simulink model "eVTOL_System"  (R2024b)
settings: Solver=FixedStepAuto  StartTime=0.0  StopTime=inf  RelTol=1e-3
undefined symbols (not defined in the file): airspeed, Battery, BCE12, BCE_Set_init, BMS_Controller_State, C, Cell10_P, Cell11_P, Cell12_P, Cell13_P, Cell14_P, Cell15_P, Cell16_P, Cell17_P, Cell18_P, Cell19_P, Cell1_N, Cell1_P, Cell20_P, Cell21_P, Cell22_P, Cell23_P, Cell24_P, Cell2_P, Cell3_P, Cell4_P, Cell5_P, Cell6_P, Cell7_P, Cell8_P, Cell9_P, Charging_State, CityMission, control, controlParams, ControlSampleTime, CriticalTiltAngle, currentFactor, CV_Gain, ddx, ddy, ddz, Device_01, Device_02, DiscIntNeverNeededParam, dx, dy, dz, Earth, env, F, F28379D_ADC_MaxCount, F28379D_ADC_Vmax, FixedWingMission, flightState, Foc_Ki_IxTcpu, Foc_Ki_S, Foc_Kp_I, Foc_Kp_S, fractalcoef ... (+68)
libraries: fl_lib x1115, nesl_utility x617, slrealtimeethercatlib x217, simulink x130, canmsglib x101, speedgoatlib_IO611_obsolete x91, slpidlib x49, mcbcontrolslib x44, slrealtimeutilitieslib x35, speedgoatlib_hdlCoder_IO3xx x31, dspstat3 x24, mcbpositiondecoderlib x12
(part 16 of 31)

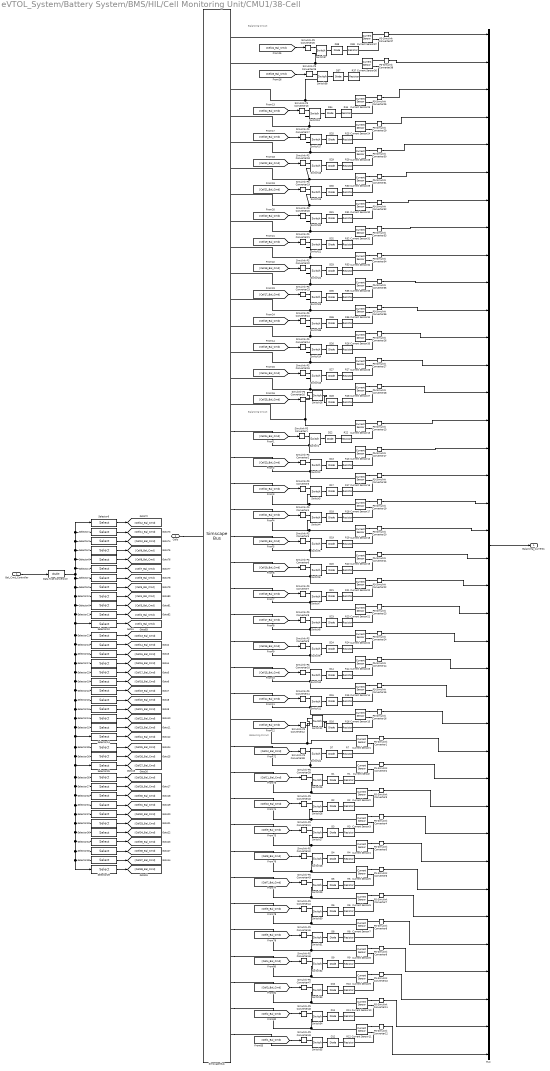
== system eVTOL_System/Battery System/BMS/HIL/Cell Monitoring Unit/CMU1/38-Cell ==
  note: Balancing Circuit
  note: Balancing Circuit
  note: Balancing Circuit
  Bal_Cmd_Controller : Inport
  Current Sensor{,1..37} (38 alike) : fl_lib/Electrical/Electrical Sensors/Current Sensor
  D{1..38} (38 alike) : fl_lib/Electrical/Electrical Elements/Diode  Vf=0.6 V  Ron=0.3 Ohm  Goff=1e-8 1/Ohm  i_specify=off  i_priority=High  i=0 A  i_nominal_specify=off  i_nominal_value=1  i_nominal_unit=A  v_specify=off  v_priority=None  v=0 V  v_nominal_specify=off  v_nominal_value=1  v_nominal_unit=V
      settings: LibrarySourceBlock=BatteryPack_lib/CellMonitoringUnit/D1  LogSimulationData=on
  Data Type Conversion : DataTypeConversion  OutDataTypeStr=double  SaturateOnIntegerOverflow=off  RndMeth=Floor
  Mux : Mux  Inputs=38
  PS-Simulink Converter{1..38} (38 alike) : nesl_utility/PS-Simulink Converter  PhysicalDomain=network_engine_domain  SubClassName=ps_output  LeftPortType=input  RightPortType=output  PseudoPeriodic=off  Frequencies=[]  VectorFormat=inherit  Unit=inherit  AffineConversion=off
  R{1..38} (38 alike) : fl_lib/Electrical/Electrical Elements/Resistor  R=Battery.R_bleed Ohm  i_specify=off  i_priority=None  i=0 A  i_nominal_specify=off  i_nominal_value=1  i_nominal_unit=A  v_specify=off  v_priority=None  v=0 V  v_nominal_specify=off  v_nominal_value=1  v_nominal_unit=V
      settings: LibrarySourceBlock=BatteryPack_lib/CellMonitoringUnit/R1  LogSimulationData=on
  Selector1 : Selector  IndexOptions=Index vector (dialog)  Indices=11  OutputSizes=1
  Selector10 : Selector  IndexOptions=Index vector (dialog)  Indices=1  OutputSizes=1
  Selector11 : Selector  IndexOptions=Index vector (dialog)  Indices=2  OutputSizes=1
  Selector12 : Selector  IndexOptions=Index vector (dialog)  Indices=4  OutputSizes=1
  Selector13 : Selector  IndexOptions=Index vector (dialog)  Indices=14  OutputSizes=1
  Selector14 : Selector  IndexOptions=Index vector (dialog)  Indices=24  OutputSizes=1
  Selector15 : Selector  IndexOptions=Index vector (dialog)  Indices=23  OutputSizes=1
  Selector16 : Selector  IndexOptions=Index vector (dialog)  Indices=21  OutputSizes=1
  Selector17 : Selector  IndexOptions=Index vector (dialog)  Indices=16  OutputSizes=1
  Selector18 : Selector  IndexOptions=Index vector (dialog)  Indices=15  OutputSizes=1
  Selector19 : Selector  IndexOptions=Index vector (dialog)  Indices=18  OutputSizes=1
  Selector2 : Selector  IndexOptions=Index vector (dialog)  Indices=9  OutputSizes=1
  Selector20 : Selector  IndexOptions=Index vector (dialog)  Indices=20  OutputSizes=1
  Selector21 : Selector  IndexOptions=Index vector (dialog)  Indices=13  OutputSizes=1
  Selector22 : Selector  IndexOptions=Index vector (dialog)  Indices=19  OutputSizes=1
  Selector23 : Selector  IndexOptions=Index vector (dialog)  Indices=17  OutputSizes=1
  Selector24 : Selector  IndexOptions=Index vector (dialog)  Indices=22  OutputSizes=1
  Selector25 : Selector  IndexOptions=Index vector (dialog)  Indices=27  OutputSizes=1
  Selector26 : Selector  IndexOptions=Index vector (dialog)  Indices=26  OutputSizes=1
  Selector27 : Selector  IndexOptions=Index vector (dialog)  Indices=29  OutputSizes=1
  Selector29 : Selector  IndexOptions=Index vector (dialog)  Indices=38  OutputSizes=1
  Selector3 : Selector  IndexOptions=Index vector (dialog)  Indices=10  OutputSizes=1
  Selector30 : Selector  IndexOptions=Index vector (dialog)  Indices=36  OutputSizes=1
  Selector31 : Selector  IndexOptions=Index vector (dialog)  Indices=31  OutputSizes=1
  Selector32 : Selector  IndexOptions=Index vector (dialog)  Indices=30  OutputSizes=1
  Selector33 : Selector  IndexOptions=Index vector (dialog)  Indices=33  OutputSizes=1
  Selector34 : Selector  IndexOptions=Index vector (dialog)  Indices=35  OutputSizes=1
  Selector35 : Selector  IndexOptions=Index vector (dialog)  Indices=28  OutputSizes=1
  Selector36 : Selector  IndexOptions=Index vector (dialog)  Indices=34  OutputSizes=1
  Selector37 : Selector  IndexOptions=Index vector (dialog)  Indices=32  OutputSizes=1
  Selector38 : Selector  IndexOptions=Index vector (dialog)  Indices=37  OutputSizes=1
  Selector39 : Selector  IndexOptions=Index vector (dialog)  Indices=25  OutputSizes=1
  Selector4 : Selector  IndexOptions=Index vector (dialog)  Indices=7  OutputSizes=1
  Selector5 : Selector  IndexOptions=Index vector (dialog)  Indices=5  OutputSizes=1
  Selector6 : Selector  IndexOptions=Index vector (dialog)  Indices=12  OutputSizes=1
  Selector7 : Selector  IndexOptions=Index vector (dialog)  Indices=6  OutputSizes=1
  Selector8 : Selector  IndexOptions=Index vector (dialog)  Indices=8  OutputSizes=1
  Selector9 : Selector  IndexOptions=Index vector (dialog)  Indices=3  OutputSizes=1
  Simscape Bus : SimscapeBus  HierarchyStrings=Cell38_P;Cell37_P;Cell36_P;Cell35_P;Cell34_P;Cell33_P;Cell32_P;Cell31_P;Cell30_P;Cell29_P;Cell28_P;Cell27_P;Cell26_P;Cell25_P;Cell24_P;Cell23_P;Cell22_P;Cell21_P;Cell20_P;Cell19_P;Cell18_P;Cell17_P;Cell16_P;Cell15_P;Cell14_P;Cell13_P;Cell12_P;Cell11_P;Cell10_P;Cell9_P;Cell8_P;Cell7_P;Cell6_P;Cell5_P;Cell4_P;Cell3_P;Cell2_P;Cell1_P;Cell1_N
  Simulink-PS Converter{1..26,38..49} (38 alike) : nesl_utility/Simulink-PS Converter  PhysicalDomain=network_engine_domain  SubClassName=ps_input  LeftPortType=input  RightPortType=output  PseudoPeriodic=off  Frequencies=[]  NoiseDistribution=none  NoiseParameters=[]  Unit=1  AffineConversion=off  FilteringAndDerivatives=zero  SimscapeFilterOrder=1  InputFilterTimeConstant=0.001  UdotUserProvided=1
      settings: LibrarySourceBlock=|
      | BatteryPack_lib/CellMonitoringUnit/Simulink-PS
      | Converter3
  Switch{1..38} (38 alike) : fl_lib/Electrical/Electrical Elements/Switch  R_closed=0.01 Ohm  G_open=1e-8 1/Ohm  Threshold=0  i_specify=off  i_priority=None  i=0 A  i_nominal_specify=off  i_nominal_value=1  i_nominal_unit=A  v_specify=off  v_priority=None  v=0 V  v_nominal_specify=off  v_nominal_value=1  v_nominal_unit=V
      settings: LibrarySourceBlock=BatteryPack_lib/CellMonitoringUnit/Switch
  Cells : PMIOPort  Side=Left
  Balancing_Currents : Outport
  wires:
  [Cell3_Bal_Cmd] -> Simulink-PS Converter47/1
  [Cell4_Bal_Cmd] -> Simulink-PS Converter46/1
  [Cell2_Bal_Cmd] -> Simulink-PS Converter48/1
  [Cell9_Bal_Cmd] -> Simulink-PS Converter41/1
  [Cell12_Bal_Cmd] -> Simulink-PS Converter38/1
  [Cell6_Bal_Cmd] -> Simulink-PS Converter44/1
  [Cell11_Bal_Cmd] -> Simulink-PS Converter39/1
  [Cell1_Bal_Cmd] -> Simulink-PS Converter49/1
  [Cell10_Bal_Cmd] -> Simulink-PS Converter40/1
  [Cell8_Bal_Cmd] -> Simulink-PS Converter42/1
  [Cell7_Bal_Cmd] -> Simulink-PS Converter43/1
  [Cell5_Bal_Cmd] -> Simulink-PS Converter45/1
  Selector11/1 -> [Cell2_Bal_Cmd]
  Selector12/1 -> [Cell4_Bal_Cmd]
  Selector3/1 -> [Cell10_Bal_Cmd]
  Selector9/1 -> [Cell3_Bal_Cmd]
  Selector1/1 -> [Cell11_Bal_Cmd]
  Selector4/1 -> [Cell7_Bal_Cmd]
  Selector8/1 -> [Cell8_Bal_Cmd]
  Selector6/1 -> [Cell12_Bal_Cmd]
  Selector7/1 -> [Cell6_Bal_Cmd]
  Selector5/1 -> [Cell5_Bal_Cmd]
  Selector10/1 -> [Cell1_Bal_Cmd]
  Selector2/1 -> [Cell9_Bal_Cmd]
  Bal_Cmd_Controller/1 -> Data Type Conversion/1
  Mux/1 -> Balancing_Currents/1
  [Cell20_Bal_Cmd] -> Simulink-PS Converter5/1
  [Cell19_Bal_Cmd] -> Simulink-PS Converter6/1
  [Cell23_Bal_Cmd] -> Simulink-PS Converter2/1
  [Cell24_Bal_Cmd] -> Simulink-PS Converter1/1
  [Cell14_Bal_Cmd] -> Simulink-PS Converter11/1
  [Cell18_Bal_Cmd] -> Simulink-PS Converter7/1
  [Cell17_Bal_Cmd] -> Simulink-PS Converter8/1
  [Cell13_Bal_Cmd] -> Simulink-PS Converter12/1
  [Cell22_Bal_Cmd] -> Simulink-PS Converter3/1
  [Cell16_Bal_Cmd] -> Simulink-PS Converter9/1
  [Cell21_Bal_Cmd] -> Simulink-PS Converter4/1
  [Cell15_Bal_Cmd] -> Simulink-PS Converter10/1
  Selector13/1 -> [Cell14_Bal_Cmd]
  Selector20/1 -> [Cell20_Bal_Cmd]
  Selector22/1 -> [Cell19_Bal_Cmd]
  Selector15/1 -> [Cell23_Bal_Cmd]
  Selector17/1 -> [Cell16_Bal_Cmd]
  Selector23/1 -> [Cell17_Bal_Cmd]
  Selector18/1 -> [Cell15_Bal_Cmd]
  Selector16/1 -> [Cell21_Bal_Cmd]
  Selector14/1 -> [Cell24_Bal_Cmd]
  Selector21/1 -> [Cell13_Bal_Cmd]
  Selector24/1 -> [Cell22_Bal_Cmd]
  Selector19/1 -> [Cell18_Bal_Cmd]
  Selector35/1 -> [Cell28_Bal_Cmd]
  Selector30/1 -> [Cell36_Bal_Cmd]
  Selector29/1 -> [Cell38_Bal_Cmd]
  Selector38/1 -> [Cell37_Bal_Cmd]
  Selector32/1 -> [Cell30_Bal_Cmd]
  Selector33/1 -> [Cell33_Bal_Cmd]
  Selector34/1 -> [Cell35_Bal_Cmd]
  Selector37/1 -> [Cell32_Bal_Cmd]
  Selector39/1 -> [Cell25_Bal_Cmd]
  Selector25/1 -> [Cell27_Bal_Cmd]
  Data Type Conversion/1 -> Selector4/1, Selector8/1, Selector2/1, Selector3/1, Selector1/1, Selector6/1, Selector7/1, Selector5/1, Selector12/1, Selector9/1, Selector11/1, Selector30/1, Selector29/1, Selector38/1, Selector34/1, Selector36/1, Selector33/1, Selector37/1, Selector31/1, Selector32/1, Selector27/1, Selector35/1, Selector25/1, Selector26/1, Selector39/1, Selector14/1, Selector15/1, Selector24/1, Selector16/1, Selector20/1, Selector22/1, Selector19/1, Selector23/1, Selector17/1, Selector18/1, Selector13/1, Selector21/1, Selector10/1
  Selector36/1 -> [Cell34_Bal_Cmd]
  Selector27/1 -> [Cell29_Bal_Cmd]
  Selector31/1 -> [Cell31_Bal_Cmd]
  Selector26/1 -> [Cell26_Bal_Cmd]
  [Cell21_Bal_Cmd] -> Simulink-PS Converter19/1
  [Cell17_Bal_Cmd] -> Simulink-PS Converter23/1
  [Cell25_Bal_Cmd] -> Simulink-PS Converter16/1
  [Cell16_Bal_Cmd] -> Simulink-PS Converter24/1
  [Cell19_Bal_Cmd] -> Simulink-PS Converter21/1
  [Cell14_Bal_Cmd] -> Simulink-PS Converter15/1
  [Cell15_Bal_Cmd] -> Simulink-PS Converter14/1
  [Cell18_Bal_Cmd] -> Simulink-PS Converter22/1
  [Cell24_Bal_Cmd] -> Simulink-PS Converter13/1
  [Cell22_Bal_Cmd] -> Simulink-PS Converter18/1
  [Cell23_Bal_Cmd] -> Simulink-PS Converter17/1
  [Cell20_Bal_Cmd] -> Simulink-PS Converter20/1
  [Cell24_Bal_Cmd] -> Simulink-PS Converter25/1
  [Cell23_Bal_Cmd] -> Simulink-PS Converter26/1
  PS-Simulink Converter37/1 -> Mux/1
  PS-Simulink Converter38/1 -> Mux/2
  PS-Simulink Converter34/1 -> Mux/9
  PS-Simulink Converter33/1 -> Mux/8
  PS-Simulink Converter35/1 -> Mux/10
  PS-Simulink Converter32/1 -> Mux/7
  PS-Simulink Converter36/1 -> Mux/11
  PS-Simulink Converter31/1 -> Mux/6
  PS-Simulink Converter26/1 -> Mux/12
  PS-Simulink Converter30/1 -> Mux/5
  PS-Simulink Converter27/1 -> Mux/13
  PS-Simulink Converter29/1 -> Mux/4
  PS-Simulink Converter28/1 -> Mux/14
  PS-Simulink Converter25/1 -> Mux/3
  PS-Simulink Converter18/1 -> Mux/17
  PS-Simulink Converter17/1 -> Mux/16
  PS-Simulink Converter19/1 -> Mux/18
  PS-Simulink Converter13/1 -> Mux/15
  PS-Simulink Converter20/1 -> Mux/19
  PS-Simulink Converter21/1 -> Mux/20
  PS-Simulink Converter22/1 -> Mux/21
  PS-Simulink Converter23/1 -> Mux/22
  PS-Simulink Converter24/1 -> Mux/23
  PS-Simulink Converter14/1 -> Mux/24
  PS-Simulink Converter15/1 -> Mux/25
  PS-Simulink Converter16/1 -> Mux/26
  PS-Simulink Converter1/1 -> Mux/27
  PS-Simulink Converter2/1 -> Mux/28
  PS-Simulink Converter3/1 -> Mux/29
  PS-Simulink Converter4/1 -> Mux/30
  PS-Simulink Converter5/1 -> Mux/31
  PS-Simulink Converter6/1 -> Mux/32
  PS-Simulink Converter7/1 -> Mux/33
  PS-Simulink Converter8/1 -> Mux/34
  PS-Simulink Converter9/1 -> Mux/35
  PS-Simulink Converter10/1 -> Mux/36
  PS-Simulink Converter11/1 -> Mux/37
  PS-Simulink Converter12/1 -> Mux/38
  connections:
  Simscape Bus/LConn32 -- Current Sensor5/LConn1 -- Switch28/RConn2
  Simscape Bus/LConn29 -- Current Sensor2/LConn1 -- Switch25/RConn2
  Simscape Bus/LConn31 -- Current Sensor4/LConn1 -- Switch27/RConn2
  Simscape Bus/LConn38 -- Current Sensor11/LConn1 -- Switch34/RConn2
  Simscape Bus/LConn30 -- Current Sensor3/LConn1 -- Switch26/RConn2
  Simscape Bus/LConn36 -- Current Sensor9/LConn1 -- Switch32/RConn2
  Simscape Bus/LConn34 -- Current Sensor7/LConn1 -- Switch30/RConn2
  Simscape Bus/LConn28 -- Current Sensor/LConn1 -- Switch24/RConn2
  Simscape Bus/LConn35 -- Current Sensor8/LConn1 -- Switch31/RConn2
  Simscape Bus/LConn33 -- Current Sensor6/LConn1 -- Switch29/RConn2
  Simscape Bus/LConn37 -- Current Sensor10/LConn1 -- Switch33/RConn2
  Simulink-PS Converter38/RConn1 -- Switch24/RConn1
  R4/RConn1 -- D4/LConn1
  Simulink-PS Converter48/RConn1 -- Switch34/RConn1
  R7/RConn1 -- D7/LConn1
  R8/RConn1 -- D8/LConn1
  Switch25/LConn1 -- D1/RConn1
  R6/RConn1 -- D6/LConn1
  R10/RConn1 -- D10/LConn1
  R12/RConn1 -- D12/LConn1
  Simulink-PS Converter49/RConn1 -- Switch35/RConn1
  R11/RConn1 -- D11/LConn1
  Switch30/LConn1 -- D6/RConn1
  Simulink-PS Converter41/RConn1 -- Switch27/RConn1
  Switch32/LConn1 -- D9/RConn1
  Switch31/LConn1 -- D8/RConn1
  Simulink-PS Converter39/RConn1 -- Switch25/RConn1
  Switch24/LConn1 -- D7/RConn1
  Simulink-PS Converter47/RConn1 -- Switch33/RConn1
  Simulink-PS Converter46/RConn1 -- Switch32/RConn1
  Switch35/LConn1 -- D12/RConn1
  Switch29/LConn1 -- D5/RConn1
  R2/RConn1 -- D2/LConn1
  Simulink-PS Converter44/RConn1 -- Switch30/RConn1
  Switch27/LConn1 -- D3/RConn1
  Switch28/LConn1 -- D4/RConn1
  Simulink-PS Converter43/RConn1 -- Switch29/RConn1
  Simulink-PS Converter45/RConn1 -- Switch31/RConn1
  R3/RConn1 -- D3/LConn1
  R9/RConn1 -- D9/LConn1
  Simulink-PS Converter42/RConn1 -- Switch28/RConn1
  Switch26/LConn1 -- D2/RConn1
  Simulink-PS Converter40/RConn1 -- Switch26/RConn1
  R5/RConn1 -- D5/LConn1
  Switch33/LConn1 -- D10/RConn1
  Switch34/LConn1 -- D11/RConn1
  R1/RConn1 -- D1/LConn1
  Simscape Bus/LConn39 -- Switch35/RConn2
  Current Sensor1/LConn1 -- Switch12/RConn2 -- Simscape Bus/LConn27
  Current Sensor1/RConn2 -- R7/LConn1
  Current Sensor2/RConn2 -- R2/LConn1
  Current Sensor3/RConn2 -- R3/LConn1
  Current Sensor4/RConn2 -- R4/LConn1
  Current Sensor5/RConn2 -- R5/LConn1
  Current Sensor6/RConn2 -- R6/LConn1
  Current Sensor7/RConn2 -- R8/LConn1
  Current Sensor8/RConn2 -- R9/LConn1
  Current Sensor9/RConn2 -- R10/LConn1
  Current Sensor10/RConn2 -- R11/LConn1
  Current Sensor11/RConn2 -- R12/LConn1
  Current Sensor/RConn2 -- R1/LConn1
  PS-Simulink Converter1/LConn1 -- Current Sensor1/RConn1
  PS-Simulink Converter2/LConn1 -- Current Sensor/RConn1
  Current Sensor2/RConn1 -- PS-Simulink Converter3/LConn1
  Current Sensor3/RConn1 -- PS-Simulink Converter4/LConn1
  PS-Simulink Converter8/LConn1 -- Current Sensor7/RConn1
  Current Sensor6/RConn1 -- PS-Simulink Converter7/LConn1
  Current Sensor5/RConn1 -- PS-Simulink Converter6/LConn1
  Current Sensor4/RConn1 -- PS-Simulink Converter5/LConn1
  Current Sensor8/RConn1 -- PS-Simulink Converter9/LConn1
  Current Sensor9/RConn1 -- PS-Simulink Converter10/LConn1
  Current Sensor10/RConn1 -- PS-Simulink Converter11/LConn1
  Current Sensor11/RConn1 -- PS-Simulink Converter12/LConn1
  Current Sensor21/LConn1 -- Simscape Bus/LConn22 -- Switch7/RConn2
  Current Sensor16/LConn1 -- Simscape Bus/LConn17 -- Switch2/RConn2
  Current Sensor17/LConn1 -- Switch3/RConn2 -- Simscape Bus/LConn18
  Current Sensor22/LConn1 -- Simscape Bus/LConn23 -- Switch8/RConn2
  Current Sensor20/LConn1 -- Simscape Bus/LConn21 -- Switch6/RConn2
  Current Sensor23/LConn1 -- Simscape Bus/LConn24 -- Switch9/RConn2
  Current Sensor14/LConn1 -- Simscape Bus/LConn25 -- Switch10/RConn2
  Current Sensor12/LConn1 -- Simscape Bus/LConn16 -- Switch1/RConn2
  Current Sensor19/LConn1 -- Simscape Bus/LConn20 -- Switch5/RConn2
  Current Sensor15/LConn1 -- Simscape Bus/LConn26 -- Switch11/RConn2
  Current Sensor18/LConn1 -- Switch4/RConn2 -- Simscape Bus/LConn19
  Current Sensor20/RConn1 -- PS-Simulink Converter22/LConn1
  Switch8/LConn1 -- D23/RConn1
  Simulink-PS Converter6/RConn1 -- Switch6/RConn1
  PS-Simulink Converter13/LConn1 -- Current Sensor13/RConn1
  Current Sensor15/RConn1 -- PS-Simulink Converter16/LConn1
  Simulink-PS Converter9/RConn1 -- Switch9/RConn1
  R17/RConn1 -- D17/LConn1
  Current Sensor18/RConn2 -- R19/LConn1
  Current Sensor12/RConn2 -- R13/LConn1
  Current Sensor19/RConn2 -- R20/LConn1
  PS-Simulink Converter17/LConn1 -- Current Sensor12/RConn1
  Simulink-PS Converter5/RConn1 -- Switch5/RConn1
  Current Sensor22/RConn2 -- R24/LConn1
  Switch7/LConn1 -- D21/RConn1
  Current Sensor13/RConn2 -- R22/LConn1
  Switch4/LConn1 -- D18/RConn1
  Current Sensor23/RConn2 -- R14/LConn1
  Current Sensor21/RConn2 -- R23/LConn1
  R19/RConn1 -- D19/LConn1
  Current Sensor14/RConn2 -- R15/LConn1
  Current Sensor22/RConn1 -- PS-Simulink Converter24/LConn1
  Simulink-PS Converter1/RConn1 -- Switch1/RConn1
  Simulink-PS Converter2/RConn1 -- Switch2/RConn1
  Switch3/LConn1 -- D17/RConn1
  Simulink-PS Converter8/RConn1 -- Switch8/RConn1
  Current Sensor23/RConn1 -- PS-Simulink Converter14/LConn1
  Switch12/LConn1 -- D16/RConn1
  Switch2/LConn1 -- D13/RConn1
  Current Sensor16/RConn2 -- R17/LConn1
  Current Sensor18/RConn1 -- PS-Simulink Converter20/LConn1
  R14/RConn1 -- D14/LConn1
  Simulink-PS Converter11/RConn1 -- Switch11/RConn1
  R20/RConn1 -- D20/LConn1
  Switch16/RConn2 -- Current Sensor13/LConn1 -- Simscape Bus/LConn15
  Current Sensor19/RConn1 -- PS-Simulink Converter21/LConn1
  R15/RConn1 -- D15/LConn1
  Simulink-PS Converter7/RConn1 -- Switch7/RConn1
  Simulink-PS Converter10/RConn1 -- Switch10/RConn1
  Current Sensor15/RConn2 -- R16/LConn1
  Switch11/LConn1 -- D15/RConn1
  Simulink-PS Converter4/RConn1 -- Switch4/RConn1
  Switch10/LConn1 -- D14/RConn1
  Current Sensor14/RConn1 -- PS-Simulink Converter15/LConn1
  Switch5/LConn1 -- D19/RConn1
  R24/RConn1 -- D24/LConn1
  R21/RConn1 -- D21/LConn1
  Current Sensor16/RConn1 -- PS-Simulink Converter18/LConn1
  R22/RConn1 -- D22/LConn1
  R18/RConn1 -- D18/LConn1
  Switch9/LConn1 -- D24/RConn1
  Switch6/LConn1 -- D20/RConn1
  PS-Simulink Converter23/LConn1 -- Current Sensor21/RConn1
  Switch1/LConn1 -- D22/RConn1
  Current Sensor20/RConn2 -- R21/LConn1
  Simulink-PS Converter3/RConn1 -- Switch3/RConn1
  R23/RConn1 -- D23/LConn1
  Simulink-PS Converter12/RConn1 -- Switch12/RConn1
  R16/RConn1 -- D16/LConn1
  R13/RConn1 -- D13/LConn1
  Current Sensor17/RConn1 -- PS-Simulink Converter19/LConn1
  Current Sensor17/RConn2 -- R18/LConn1
  Cells/RConn1 -- Simscape Bus/RConn1
  Switch20/RConn2 -- Simscape Bus/LConn8 -- Current Sensor31/LConn1
  Switch14/RConn2 -- Simscape Bus/LConn13 -- Current Sensor26/LConn1
  Switch19/RConn2 -- Simscape Bus/LConn7 -- Current Sensor30/LConn1
  Switch36/RConn2 -- Simscape Bus/LConn12 -- Current Sensor35/LConn1
  Switch21/RConn2 -- Simscape Bus/LConn9 -- Current Sensor32/LConn1
  Switch15/RConn2 -- Simscape Bus/LConn14 -- Current Sensor27/LConn1
  Switch22/RConn2 -- Simscape Bus/LConn10 -- Current Sensor33/LConn1
  Switch18/RConn2 -- Simscape Bus/LConn6 -- Current Sensor29/LConn1
  Switch23/RConn2 -- Simscape Bus/LConn11 -- Current Sensor34/LConn1
  Switch17/RConn2 -- Simscape Bus/LConn5 -- Current Sensor28/LConn1
  Switch13/RConn2 -- Simscape Bus/LConn4 -- Current Sensor24/LConn1
  Switch13/LConn1 -- D34/RConn1
  Switch36/LConn1 -- D36/RConn1
  Simulink-PS Converter23/RConn1 -- Switch23/RConn1
  Switch16/LConn1 -- D28/RConn1
  Current Sensor27/RConn1 -- PS-Simulink Converter28/LConn1
  Current Sensor29/RConn2 -- R30/LConn1
  Current Sensor34/RConn1 -- PS-Simulink Converter36/LConn1
  Simulink-PS Converter20/RConn1 -- Switch20/RConn1
  R31/RConn1 -- D31/LConn1
  R25/RConn1 -- D25/LConn1
  Current Sensor31/RConn2 -- R32/LConn1
  Simulink-PS Converter18/RConn1 -- Switch18/RConn1
  Current Sensor26/RConn2 -- R27/LConn1
  Current Sensor31/RConn1 -- PS-Simulink Converter33/LConn1
  R30/RConn1 -- D30/LConn1
  Current Sensor26/RConn1 -- PS-Simulink Converter27/LConn1
  Current Sensor30/RConn2 -- R31/LConn1
  Current Sensor27/RConn2 -- R28/LConn1
  Current Sensor32/RConn2 -- R33/LConn1
  Switch20/LConn1 -- D31/RConn1
  Simulink-PS Converter22/RConn1 -- Switch22/RConn1
  Simulink-PS Converter15/RConn1 -- Switch15/RConn1
  PS-Simulink Converter29/LConn1 -- Current Sensor24/RConn1
  R32/RConn1 -- D32/LConn1
  Simulink-PS Converter17/RConn1 -- Switch17/RConn1
  Current Sensor30/RConn1 -- PS-Simulink Converter32/LConn1
  Switch14/LConn1 -- D26/RConn1
  Switch17/LConn1 -- D25/RConn1
  R35/RConn1 -- D35/LConn1
  R27/RConn1 -- D27/LConn1
  Simulink-PS Converter21/RConn1 -- Switch21/RConn1
  Switch22/LConn1 -- D33/RConn1
  Simulink-PS Converter14/RConn1 -- Switch14/RConn1
  Simulink-PS Converter19/RConn1 -- Switch19/RConn1
  R36/RConn1 -- D36/LConn1
  Current Sensor34/RConn2 -- R36/LConn1
  PS-Simulink Converter35/LConn1 -- Current Sensor33/RConn1
  Current Sensor25/LConn1 -- Switch38/RConn2 -- Simscape Bus/LConn3
  Switch23/LConn1 -- D35/RConn1
  PS-Simulink Converter25/LConn1 -- Current Sensor25/RConn1
  Simulink-PS Converter13/RConn1 -- Switch13/RConn1
  R26/RConn1 -- D26/LConn1
  R28/RConn1 -- D28/LConn1
  Simulink-PS Converter16/RConn1 -- Switch16/RConn1
  Switch18/LConn1 -- D29/RConn1
  Current Sensor35/RConn2 -- R26/LConn1
  R33/RConn1 -- D33/LConn1
  Current Sensor28/RConn1 -- PS-Simulink Converter30/LConn1
  Current Sensor24/RConn2 -- R25/LConn1
  Current Sensor32/RConn1 -- PS-Simulink Converter34/LConn1
  Current Sensor28/RConn2 -- R29/LConn1
  R34/RConn1 -- D34/LConn1
  Switch19/LConn1 -- D30/RConn1
  Simulink-PS Converter24/RConn1 -- Switch36/RConn1
  Switch21/LConn1 -- D32/RConn1
  Switch15/LConn1 -- D27/RConn1
  Current Sensor33/RConn2 -- R35/LConn1
  R29/RConn1 -- D29/LConn1
  Current Sensor29/RConn1 -- PS-Simulink Converter31/LConn1
  Current Sensor35/RConn1 -- PS-Simulink Converter26/LConn1
  Current Sensor25/RConn2 -- R34/LConn1
  Switch37/RConn2 -- Simscape Bus/LConn2 -- Current Sensor36/LConn1
  Switch38/LConn1 -- D37/RConn1
  R38/RConn1 -- D38/LConn1
  PS-Simulink Converter37/LConn1 -- Current Sensor37/RConn1
  R37/RConn1 -- D37/LConn1
  Current Sensor36/RConn2 -- R37/LConn1
  Switch37/LConn1 -- D38/RConn1
  Current Sensor37/LConn1 -- Simscape Bus/LConn1
  Simulink-PS Converter26/RConn1 -- Switch38/RConn1
  PS-Simulink Converter38/LConn1 -- Current Sensor36/RConn1
  Simulink-PS Converter25/RConn1 -- Switch37/RConn1
  Current Sensor37/RConn2 -- R38/LConn1

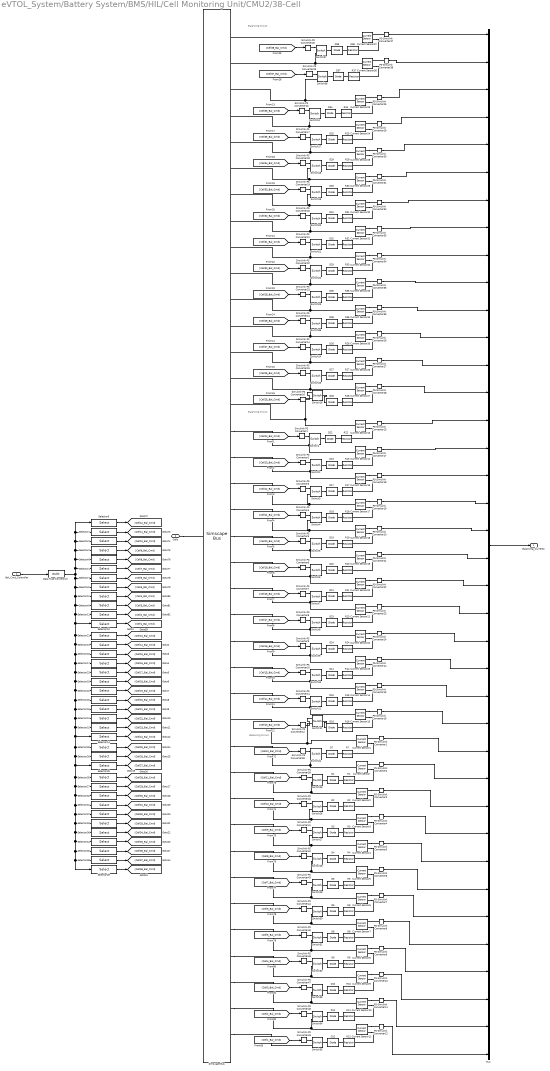
== system eVTOL_System/Battery System/BMS/HIL/Cell Monitoring Unit/CMU2/38-Cell ==
  note: Balancing Circuit
  note: Balancing Circuit
  note: Balancing Circuit
  Bal_Cmd_Controller : Inport
  Current Sensor{,1..37} (38 alike) : fl_lib/Electrical/Electrical Sensors/Current Sensor
  D{1..38} (38 alike) : fl_lib/Electrical/Electrical Elements/Diode  Vf=0.6 V  Ron=0.3 Ohm  Goff=1e-8 1/Ohm  i_specify=off  i_priority=High  i=0 A  i_nominal_specify=off  i_nominal_value=1  i_nominal_unit=A  v_specify=off  v_priority=None  v=0 V  v_nominal_specify=off  v_nominal_value=1  v_nominal_unit=V
      settings: LibrarySourceBlock=BatteryPack_lib/CellMonitoringUnit/D1  LogSimulationData=on
  Data Type Conversion : DataTypeConversion  OutDataTypeStr=double  SaturateOnIntegerOverflow=off  RndMeth=Floor
  Mux : Mux  Inputs=38
  PS-Simulink Converter{1..38} (38 alike) : nesl_utility/PS-Simulink Converter  PhysicalDomain=network_engine_domain  SubClassName=ps_output  LeftPortType=input  RightPortType=output  PseudoPeriodic=off  Frequencies=[]  VectorFormat=inherit  Unit=inherit  AffineConversion=off
  R{1..38} (38 alike) : fl_lib/Electrical/Electrical Elements/Resistor  R=Battery.R_bleed Ohm  i_specify=off  i_priority=None  i=0 A  i_nominal_specify=off  i_nominal_value=1  i_nominal_unit=A  v_specify=off  v_priority=None  v=0 V  v_nominal_specify=off  v_nominal_value=1  v_nominal_unit=V
      settings: LibrarySourceBlock=BatteryPack_lib/CellMonitoringUnit/R1  LogSimulationData=on
  Selector1 : Selector  IndexOptions=Index vector (dialog)  Indices=49  OutputSizes=1
  Selector10 : Selector  IndexOptions=Index vector (dialog)  Indices=39  OutputSizes=1
  Selector11 : Selector  IndexOptions=Index vector (dialog)  Indices=40  OutputSizes=1
  Selector12 : Selector  IndexOptions=Index vector (dialog)  Indices=42  OutputSizes=1
  Selector13 : Selector  IndexOptions=Index vector (dialog)  Indices=52  OutputSizes=1
  Selector14 : Selector  IndexOptions=Index vector (dialog)  Indices=62  OutputSizes=1
  Selector15 : Selector  IndexOptions=Index vector (dialog)  Indices=61  OutputSizes=1
  Selector16 : Selector  IndexOptions=Index vector (dialog)  Indices=59  OutputSizes=1
  Selector17 : Selector  IndexOptions=Index vector (dialog)  Indices=54  OutputSizes=1
  Selector18 : Selector  IndexOptions=Index vector (dialog)  Indices=53  OutputSizes=1
  Selector19 : Selector  IndexOptions=Index vector (dialog)  Indices=56  OutputSizes=1
  Selector2 : Selector  IndexOptions=Index vector (dialog)  Indices=47  OutputSizes=1
  Selector20 : Selector  IndexOptions=Index vector (dialog)  Indices=58  OutputSizes=1
  Selector21 : Selector  IndexOptions=Index vector (dialog)  Indices=51  OutputSizes=1
  Selector22 : Selector  IndexOptions=Index vector (dialog)  Indices=57  OutputSizes=1
  Selector23 : Selector  IndexOptions=Index vector (dialog)  Indices=55  OutputSizes=1
  Selector24 : Selector  IndexOptions=Index vector (dialog)  Indices=60  OutputSizes=1
  Selector25 : Selector  IndexOptions=Index vector (dialog)  Indices=65  OutputSizes=1
  Selector26 : Selector  IndexOptions=Index vector (dialog)  Indices=64  OutputSizes=1
  Selector27 : Selector  IndexOptions=Index vector (dialog)  Indices=67  OutputSizes=1
  Selector29 : Selector  IndexOptions=Index vector (dialog)  Indices=76  OutputSizes=1
  Selector3 : Selector  IndexOptions=Index vector (dialog)  Indices=48  OutputSizes=1
  Selector30 : Selector  IndexOptions=Index vector (dialog)  Indices=74  OutputSizes=1
  Selector31 : Selector  IndexOptions=Index vector (dialog)  Indices=69  OutputSizes=1
  Selector32 : Selector  IndexOptions=Index vector (dialog)  Indices=68  OutputSizes=1
  Selector33 : Selector  IndexOptions=Index vector (dialog)  Indices=71  OutputSizes=1
  Selector34 : Selector  IndexOptions=Index vector (dialog)  Indices=73  OutputSizes=1
  Selector35 : Selector  IndexOptions=Index vector (dialog)  Indices=66  OutputSizes=1
  Selector36 : Selector  IndexOptions=Index vector (dialog)  Indices=72  OutputSizes=1
  Selector37 : Selector  IndexOptions=Index vector (dialog)  Indices=70  OutputSizes=1
  Selector38 : Selector  IndexOptions=Index vector (dialog)  Indices=75  OutputSizes=1
  Selector39 : Selector  IndexOptions=Index vector (dialog)  Indices=63  OutputSizes=1
  Selector4 : Selector  IndexOptions=Index vector (dialog)  Indices=45  OutputSizes=1
  Selector5 : Selector  IndexOptions=Index vector (dialog)  Indices=43  OutputSizes=1
  Selector6 : Selector  IndexOptions=Index vector (dialog)  Indices=50  OutputSizes=1
  Selector7 : Selector  IndexOptions=Index vector (dialog)  Indices=44  OutputSizes=1
  Selector8 : Selector  IndexOptions=Index vector (dialog)  Indices=46  OutputSizes=1
  Selector9 : Selector  IndexOptions=Index vector (dialog)  Indices=41  OutputSizes=1
  Simscape Bus : SimscapeBus  HierarchyStrings=Cell38_P;Cell37_P;Cell36_P;Cell35_P;Cell34_P;Cell33_P;Cell32_P;Cell31_P;Cell30_P;Cell29_P;Cell28_P;Cell27_P;Cell26_P;Cell25_P;Cell24_P;Cell23_P;Cell22_P;Cell21_P;Cell20_P;Cell19_P;Cell18_P;Cell17_P;Cell16_P;Cell15_P;Cell14_P;Cell13_P;Cell12_P;Cell11_P;Cell10_P;Cell9_P;Cell8_P;Cell7_P;Cell6_P;Cell5_P;Cell4_P;Cell3_P;Cell2_P;Cell1_P;Cell1_N
  Simulink-PS Converter{1..26,38..49} (38 alike) : nesl_utility/Simulink-PS Converter  PhysicalDomain=network_engine_domain  SubClassName=ps_input  LeftPortType=input  RightPortType=output  PseudoPeriodic=off  Frequencies=[]  NoiseDistribution=none  NoiseParameters=[]  Unit=1  AffineConversion=off  FilteringAndDerivatives=zero  SimscapeFilterOrder=1  InputFilterTimeConstant=0.001  UdotUserProvided=1
      settings: LibrarySourceBlock=|
      | BatteryPack_lib/CellMonitoringUnit/Simulink-PS
      | Converter3
  Switch{1..38} (38 alike) : fl_lib/Electrical/Electrical Elements/Switch  R_closed=0.01 Ohm  G_open=1e-8 1/Ohm  Threshold=0  i_specify=off  i_priority=None  i=0 A  i_nominal_specify=off  i_nominal_value=1  i_nominal_unit=A  v_specify=off  v_priority=None  v=0 V  v_nominal_specify=off  v_nominal_value=1  v_nominal_unit=V
      settings: LibrarySourceBlock=BatteryPack_lib/CellMonitoringUnit/Switch
  Cells : PMIOPort  Side=Left
  Balancing_Currents : Outport
  wires:
  [Cell3_Bal_Cmd] -> Simulink-PS Converter47/1
  [Cell4_Bal_Cmd] -> Simulink-PS Converter46/1
  [Cell2_Bal_Cmd] -> Simulink-PS Converter48/1
  [Cell9_Bal_Cmd] -> Simulink-PS Converter41/1
  [Cell12_Bal_Cmd] -> Simulink-PS Converter38/1
  [Cell6_Bal_Cmd] -> Simulink-PS Converter44/1
  [Cell11_Bal_Cmd] -> Simulink-PS Converter39/1
  [Cell1_Bal_Cmd] -> Simulink-PS Converter49/1
  [Cell10_Bal_Cmd] -> Simulink-PS Converter40/1
  [Cell8_Bal_Cmd] -> Simulink-PS Converter42/1
  [Cell7_Bal_Cmd] -> Simulink-PS Converter43/1
  [Cell5_Bal_Cmd] -> Simulink-PS Converter45/1
  Selector11/1 -> [Cell2_Bal_Cmd]
  Selector12/1 -> [Cell4_Bal_Cmd]
  Selector3/1 -> [Cell10_Bal_Cmd]
  Selector9/1 -> [Cell3_Bal_Cmd]
  Selector1/1 -> [Cell11_Bal_Cmd]
  Selector4/1 -> [Cell7_Bal_Cmd]
  Selector8/1 -> [Cell8_Bal_Cmd]
  Selector6/1 -> [Cell12_Bal_Cmd]
  Selector7/1 -> [Cell6_Bal_Cmd]
  Selector5/1 -> [Cell5_Bal_Cmd]
  Selector10/1 -> [Cell1_Bal_Cmd]
  Selector2/1 -> [Cell9_Bal_Cmd]
  Bal_Cmd_Controller/1 -> Data Type Conversion/1
  Mux/1 -> Balancing_Currents/1
  [Cell20_Bal_Cmd] -> Simulink-PS Converter5/1
  [Cell19_Bal_Cmd] -> Simulink-PS Converter6/1
  [Cell23_Bal_Cmd] -> Simulink-PS Converter2/1
  [Cell24_Bal_Cmd] -> Simulink-PS Converter1/1
  [Cell14_Bal_Cmd] -> Simulink-PS Converter11/1
  [Cell18_Bal_Cmd] -> Simulink-PS Converter7/1
  [Cell17_Bal_Cmd] -> Simulink-PS Converter8/1
  [Cell13_Bal_Cmd] -> Simulink-PS Converter12/1
  [Cell22_Bal_Cmd] -> Simulink-PS Converter3/1
  [Cell16_Bal_Cmd] -> Simulink-PS Converter9/1
  [Cell21_Bal_Cmd] -> Simulink-PS Converter4/1
  [Cell15_Bal_Cmd] -> Simulink-PS Converter10/1
  Selector13/1 -> [Cell14_Bal_Cmd]
  Selector20/1 -> [Cell20_Bal_Cmd]
  Selector22/1 -> [Cell19_Bal_Cmd]
  Selector15/1 -> [Cell23_Bal_Cmd]
  Selector17/1 -> [Cell16_Bal_Cmd]
  Selector23/1 -> [Cell17_Bal_Cmd]
  Selector18/1 -> [Cell15_Bal_Cmd]
  Selector16/1 -> [Cell21_Bal_Cmd]
  Selector14/1 -> [Cell24_Bal_Cmd]
  Selector21/1 -> [Cell13_Bal_Cmd]
  Selector24/1 -> [Cell22_Bal_Cmd]
  Selector19/1 -> [Cell18_Bal_Cmd]
  Selector35/1 -> [Cell28_Bal_Cmd]
  Selector30/1 -> [Cell36_Bal_Cmd]
  Selector29/1 -> [Cell38_Bal_Cmd]
  Selector38/1 -> [Cell37_Bal_Cmd]
  Selector32/1 -> [Cell30_Bal_Cmd]
  Selector33/1 -> [Cell33_Bal_Cmd]
  Selector34/1 -> [Cell35_Bal_Cmd]
  Selector37/1 -> [Cell32_Bal_Cmd]
  Selector39/1 -> [Cell25_Bal_Cmd]
  Selector25/1 -> [Cell27_Bal_Cmd]
  Data Type Conversion/1 -> Selector4/1, Selector8/1, Selector2/1, Selector3/1, Selector1/1, Selector6/1, Selector7/1, Selector5/1, Selector12/1, Selector9/1, Selector11/1, Selector30/1, Selector29/1, Selector38/1, Selector34/1, Selector36/1, Selector33/1, Selector37/1, Selector31/1, Selector32/1, Selector27/1, Selector35/1, Selector25/1, Selector26/1, Selector39/1, Selector14/1, Selector15/1, Selector24/1, Selector16/1, Selector20/1, Selector22/1, Selector19/1, Selector23/1, Selector17/1, Selector18/1, Selector13/1, Selector21/1, Selector10/1
  Selector36/1 -> [Cell34_Bal_Cmd]
  Selector27/1 -> [Cell29_Bal_Cmd]
  Selector31/1 -> [Cell31_Bal_Cmd]
  Selector26/1 -> [Cell26_Bal_Cmd]
  [Cell33_Bal_Cmd] -> Simulink-PS Converter19/1
  [Cell29_Bal_Cmd] -> Simulink-PS Converter23/1
  [Cell25_Bal_Cmd] -> Simulink-PS Converter16/1
  [Cell28_Bal_Cmd] -> Simulink-PS Converter24/1
  [Cell31_Bal_Cmd] -> Simulink-PS Converter21/1
  [Cell26_Bal_Cmd] -> Simulink-PS Converter15/1
  [Cell27_Bal_Cmd] -> Simulink-PS Converter14/1
  [Cell30_Bal_Cmd] -> Simulink-PS Converter22/1
  [Cell36_Bal_Cmd] -> Simulink-PS Converter13/1
  [Cell34_Bal_Cmd] -> Simulink-PS Converter18/1
  [Cell35_Bal_Cmd] -> Simulink-PS Converter17/1
  [Cell32_Bal_Cmd] -> Simulink-PS Converter20/1
  [Cell38_Bal_Cmd] -> Simulink-PS Converter25/1
  [Cell37_Bal_Cmd] -> Simulink-PS Converter26/1
  PS-Simulink Converter37/1 -> Mux/1
  PS-Simulink Converter38/1 -> Mux/2
  PS-Simulink Converter34/1 -> Mux/9
  PS-Simulink Converter33/1 -> Mux/8
  PS-Simulink Converter35/1 -> Mux/10
  PS-Simulink Converter32/1 -> Mux/7
  PS-Simulink Converter36/1 -> Mux/11
  PS-Simulink Converter31/1 -> Mux/6
  PS-Simulink Converter26/1 -> Mux/12
  PS-Simulink Converter30/1 -> Mux/5
  PS-Simulink Converter27/1 -> Mux/13
  PS-Simulink Converter29/1 -> Mux/4
  PS-Simulink Converter28/1 -> Mux/14
  PS-Simulink Converter25/1 -> Mux/3
  PS-Simulink Converter18/1 -> Mux/17
  PS-Simulink Converter17/1 -> Mux/16
  PS-Simulink Converter19/1 -> Mux/18
  PS-Simulink Converter13/1 -> Mux/15
  PS-Simulink Converter20/1 -> Mux/19
  PS-Simulink Converter21/1 -> Mux/20
  PS-Simulink Converter22/1 -> Mux/21
  PS-Simulink Converter23/1 -> Mux/22
  PS-Simulink Converter24/1 -> Mux/23
  PS-Simulink Converter14/1 -> Mux/24
  PS-Simulink Converter15/1 -> Mux/25
  PS-Simulink Converter16/1 -> Mux/26
  PS-Simulink Converter1/1 -> Mux/27
  PS-Simulink Converter2/1 -> Mux/28
  PS-Simulink Converter3/1 -> Mux/29
  PS-Simulink Converter4/1 -> Mux/30
  PS-Simulink Converter5/1 -> Mux/31
  PS-Simulink Converter6/1 -> Mux/32
  PS-Simulink Converter7/1 -> Mux/33
  PS-Simulink Converter8/1 -> Mux/34
  PS-Simulink Converter9/1 -> Mux/35
  PS-Simulink Converter10/1 -> Mux/36
  PS-Simulink Converter11/1 -> Mux/37
  PS-Simulink Converter12/1 -> Mux/38
  connections:
  Current Sensor5/LConn1 -- Simscape Bus/LConn32 -- Switch28/RConn2
  Current Sensor2/LConn1 -- Simscape Bus/LConn29 -- Switch25/RConn2
  Simscape Bus/LConn31 -- Current Sensor4/LConn1 -- Switch27/RConn2
  Current Sensor11/LConn1 -- Simscape Bus/LConn38 -- Switch34/RConn2
  Simscape Bus/LConn30 -- Current Sensor3/LConn1 -- Switch26/RConn2
  Current Sensor9/LConn1 -- Simscape Bus/LConn36 -- Switch32/RConn2
  Current Sensor7/LConn1 -- Simscape Bus/LConn34 -- Switch30/RConn2
  Current Sensor/LConn1 -- Simscape Bus/LConn28 -- Switch24/RConn2
  Current Sensor8/LConn1 -- Simscape Bus/LConn35 -- Switch31/RConn2
  Current Sensor6/LConn1 -- Simscape Bus/LConn33 -- Switch29/RConn2
  Current Sensor10/LConn1 -- Simscape Bus/LConn37 -- Switch33/RConn2
  Simulink-PS Converter38/RConn1 -- Switch24/RConn1
  R4/RConn1 -- D4/LConn1
  Simulink-PS Converter48/RConn1 -- Switch34/RConn1
  R7/RConn1 -- D7/LConn1
  R8/RConn1 -- D8/LConn1
  Switch25/LConn1 -- D1/RConn1
  R6/RConn1 -- D6/LConn1
  R10/RConn1 -- D10/LConn1
  R12/RConn1 -- D12/LConn1
  Simulink-PS Converter49/RConn1 -- Switch35/RConn1
  R11/RConn1 -- D11/LConn1
  Switch30/LConn1 -- D6/RConn1
  Simulink-PS Converter41/RConn1 -- Switch27/RConn1
  Switch32/LConn1 -- D9/RConn1
  Switch31/LConn1 -- D8/RConn1
  Simulink-PS Converter39/RConn1 -- Switch25/RConn1
  Switch24/LConn1 -- D7/RConn1
  Simulink-PS Converter47/RConn1 -- Switch33/RConn1
  Simulink-PS Converter46/RConn1 -- Switch32/RConn1
  Switch35/LConn1 -- D12/RConn1
  Switch29/LConn1 -- D5/RConn1
  R2/RConn1 -- D2/LConn1
  Simulink-PS Converter44/RConn1 -- Switch30/RConn1
  Switch27/LConn1 -- D3/RConn1
  Switch28/LConn1 -- D4/RConn1
  Simulink-PS Converter43/RConn1 -- Switch29/RConn1
  Simulink-PS Converter45/RConn1 -- Switch31/RConn1
  R3/RConn1 -- D3/LConn1
  R9/RConn1 -- D9/LConn1
  Simulink-PS Converter42/RConn1 -- Switch28/RConn1
  Switch26/LConn1 -- D2/RConn1
  Simulink-PS Converter40/RConn1 -- Switch26/RConn1
  R5/RConn1 -- D5/LConn1
  Switch33/LConn1 -- D10/RConn1
  Switch34/LConn1 -- D11/RConn1
  R1/RConn1 -- D1/LConn1
  Simscape Bus/LConn39 -- Switch35/RConn2
  Current Sensor1/LConn1 -- Switch12/RConn2 -- Simscape Bus/LConn27
  Current Sensor1/RConn2 -- R7/LConn1
  Current Sensor2/RConn2 -- R2/LConn1
  Current Sensor3/RConn2 -- R3/LConn1
  Current Sensor4/RConn2 -- R4/LConn1
  Current Sensor5/RConn2 -- R5/LConn1
  Current Sensor6/RConn2 -- R6/LConn1
  Current Sensor7/RConn2 -- R8/LConn1
  Current Sensor8/RConn2 -- R9/LConn1
  Current Sensor9/RConn2 -- R10/LConn1
  Current Sensor10/RConn2 -- R11/LConn1
  Current Sensor11/RConn2 -- R12/LConn1
  Current Sensor/RConn2 -- R1/LConn1
  PS-Simulink Converter1/LConn1 -- Current Sensor1/RConn1
  PS-Simulink Converter2/LConn1 -- Current Sensor/RConn1
  Current Sensor2/RConn1 -- PS-Simulink Converter3/LConn1
  Current Sensor3/RConn1 -- PS-Simulink Converter4/LConn1
  PS-Simulink Converter8/LConn1 -- Current Sensor7/RConn1
  Current Sensor6/RConn1 -- PS-Simulink Converter7/LConn1
  Current Sensor5/RConn1 -- PS-Simulink Converter6/LConn1
  Current Sensor4/RConn1 -- PS-Simulink Converter5/LConn1
  Current Sensor8/RConn1 -- PS-Simulink Converter9/LConn1
  Current Sensor9/RConn1 -- PS-Simulink Converter10/LConn1
  Current Sensor10/RConn1 -- PS-Simulink Converter11/LConn1
  Current Sensor11/RConn1 -- PS-Simulink Converter12/LConn1
  Current Sensor21/LConn1 -- Switch7/RConn2 -- Simscape Bus/LConn22
  Current Sensor16/LConn1 -- Switch2/RConn2 -- Simscape Bus/LConn17
  Current Sensor17/LConn1 -- Switch3/RConn2 -- Simscape Bus/LConn18
  Current Sensor22/LConn1 -- Switch8/RConn2 -- Simscape Bus/LConn23
  Current Sensor20/LConn1 -- Switch6/RConn2 -- Simscape Bus/LConn21
  Current Sensor23/LConn1 -- Switch9/RConn2 -- Simscape Bus/LConn24
  Current Sensor14/LConn1 -- Switch10/RConn2 -- Simscape Bus/LConn25
  Current Sensor12/LConn1 -- Switch1/RConn2 -- Simscape Bus/LConn16
  Current Sensor19/LConn1 -- Switch5/RConn2 -- Simscape Bus/LConn20
  Current Sensor15/LConn1 -- Switch11/RConn2 -- Simscape Bus/LConn26
  Current Sensor18/LConn1 -- Switch4/RConn2 -- Simscape Bus/LConn19
  Current Sensor20/RConn1 -- PS-Simulink Converter22/LConn1
  Switch8/LConn1 -- D23/RConn1
  Simulink-PS Converter6/RConn1 -- Switch6/RConn1
  PS-Simulink Converter13/LConn1 -- Current Sensor13/RConn1
  Current Sensor15/RConn1 -- PS-Simulink Converter16/LConn1
  Simulink-PS Converter9/RConn1 -- Switch9/RConn1
  R17/RConn1 -- D17/LConn1
  Current Sensor18/RConn2 -- R19/LConn1
  Current Sensor12/RConn2 -- R13/LConn1
  Current Sensor19/RConn2 -- R20/LConn1
  PS-Simulink Converter17/LConn1 -- Current Sensor12/RConn1
  Simulink-PS Converter5/RConn1 -- Switch5/RConn1
  Current Sensor22/RConn2 -- R24/LConn1
  Switch7/LConn1 -- D21/RConn1
  Current Sensor13/RConn2 -- R22/LConn1
  Switch4/LConn1 -- D18/RConn1
  Current Sensor23/RConn2 -- R14/LConn1
  Current Sensor21/RConn2 -- R23/LConn1
  R19/RConn1 -- D19/LConn1
  Current Sensor14/RConn2 -- R15/LConn1
  Current Sensor22/RConn1 -- PS-Simulink Converter24/LConn1
  Simulink-PS Converter1/RConn1 -- Switch1/RConn1
  Simulink-PS Converter2/RConn1 -- Switch2/RConn1
  Switch3/LConn1 -- D17/RConn1
  Simulink-PS Converter8/RConn1 -- Switch8/RConn1
  Current Sensor23/RConn1 -- PS-Simulink Converter14/LConn1
  Switch12/LConn1 -- D16/RConn1
  Switch2/LConn1 -- D13/RConn1
  Current Sensor16/RConn2 -- R17/LConn1
  Current Sensor18/RConn1 -- PS-Simulink Converter20/LConn1
  R14/RConn1 -- D14/LConn1
  Simulink-PS Converter11/RConn1 -- Switch11/RConn1
  R20/RConn1 -- D20/LConn1
  Switch16/RConn2 -- Simscape Bus/LConn15 -- Current Sensor13/LConn1
  Current Sensor19/RConn1 -- PS-Simulink Converter21/LConn1
  R15/RConn1 -- D15/LConn1
  Simulink-PS Converter7/RConn1 -- Switch7/RConn1
  Simulink-PS Converter10/RConn1 -- Switch10/RConn1
  Current Sensor15/RConn2 -- R16/LConn1
  Switch11/LConn1 -- D15/RConn1
  Simulink-PS Converter4/RConn1 -- Switch4/RConn1
  Switch10/LConn1 -- D14/RConn1
  Current Sensor14/RConn1 -- PS-Simulink Converter15/LConn1
  Switch5/LConn1 -- D19/RConn1
  R24/RConn1 -- D24/LConn1
  R21/RConn1 -- D21/LConn1
  Current Sensor16/RConn1 -- PS-Simulink Converter18/LConn1
  R22/RConn1 -- D22/LConn1
  R18/RConn1 -- D18/LConn1
  Switch9/LConn1 -- D24/RConn1
  Switch6/LConn1 -- D20/RConn1
  PS-Simulink Converter23/LConn1 -- Current Sensor21/RConn1
  Switch1/LConn1 -- D22/RConn1
  Current Sensor20/RConn2 -- R21/LConn1
  Simulink-PS Converter3/RConn1 -- Switch3/RConn1
  R23/RConn1 -- D23/LConn1
  Simulink-PS Converter12/RConn1 -- Switch12/RConn1
  R16/RConn1 -- D16/LConn1
  R13/RConn1 -- D13/LConn1
  Current Sensor17/RConn1 -- PS-Simulink Converter19/LConn1
  Current Sensor17/RConn2 -- R18/LConn1
  Cells/RConn1 -- Simscape Bus/RConn1
  Current Sensor31/LConn1 -- Switch20/RConn2 -- Simscape Bus/LConn8
  Current Sensor26/LConn1 -- Switch14/RConn2 -- Simscape Bus/LConn13
  Current Sensor30/LConn1 -- Switch19/RConn2 -- Simscape Bus/LConn7
  Current Sensor35/LConn1 -- Switch36/RConn2 -- Simscape Bus/LConn12
  Current Sensor32/LConn1 -- Switch21/RConn2 -- Simscape Bus/LConn9
  Current Sensor27/LConn1 -- Switch15/RConn2 -- Simscape Bus/LConn14
  Current Sensor33/LConn1 -- Switch22/RConn2 -- Simscape Bus/LConn10
  Current Sensor29/LConn1 -- Switch18/RConn2 -- Simscape Bus/LConn6
  Current Sensor34/LConn1 -- Switch23/RConn2 -- Simscape Bus/LConn11
  Current Sensor28/LConn1 -- Switch17/RConn2 -- Simscape Bus/LConn5
  Current Sensor24/LConn1 -- Switch13/RConn2 -- Simscape Bus/LConn4
  Switch13/LConn1 -- D34/RConn1
  Switch36/LConn1 -- D36/RConn1
  Simulink-PS Converter23/RConn1 -- Switch23/RConn1
  Switch16/LConn1 -- D28/RConn1
  Current Sensor27/RConn1 -- PS-Simulink Converter28/LConn1
  Current Sensor29/RConn2 -- R30/LConn1
  Current Sensor34/RConn1 -- PS-Simulink Converter36/LConn1
  Simulink-PS Converter20/RConn1 -- Switch20/RConn1
  R31/RConn1 -- D31/LConn1
  R25/RConn1 -- D25/LConn1
  Current Sensor31/RConn2 -- R32/LConn1
  Simulink-PS Converter18/RConn1 -- Switch18/RConn1
  Current Sensor26/RConn2 -- R27/LConn1
  Current Sensor31/RConn1 -- PS-Simulink Converter33/LConn1
  R30/RConn1 -- D30/LConn1
  Current Sensor26/RConn1 -- PS-Simulink Converter27/LConn1
  Current Sensor30/RConn2 -- R31/LConn1
  Current Sensor27/RConn2 -- R28/LConn1
  Current Sensor32/RConn2 -- R33/LConn1
  Switch20/LConn1 -- D31/RConn1
  Simulink-PS Converter22/RConn1 -- Switch22/RConn1
  Simulink-PS Converter15/RConn1 -- Switch15/RConn1
  PS-Simulink Converter29/LConn1 -- Current Sensor24/RConn1
  R32/RConn1 -- D32/LConn1
  Simulink-PS Converter17/RConn1 -- Switch17/RConn1
  Current Sensor30/RConn1 -- PS-Simulink Converter32/LConn1
  Switch14/LConn1 -- D26/RConn1
  Switch17/LConn1 -- D25/RConn1
  R35/RConn1 -- D35/LConn1
  R27/RConn1 -- D27/LConn1
  Simulink-PS Converter21/RConn1 -- Switch21/RConn1
  Switch22/LConn1 -- D33/RConn1
  Simulink-PS Converter14/RConn1 -- Switch14/RConn1
  Simulink-PS Converter19/RConn1 -- Switch19/RConn1
  R36/RConn1 -- D36/LConn1
  Current Sensor34/RConn2 -- R36/LConn1
  PS-Simulink Converter35/LConn1 -- Current Sensor33/RConn1
  Simscape Bus/LConn3 -- Current Sensor25/LConn1 -- Switch38/RConn2
  Switch23/LConn1 -- D35/RConn1
  PS-Simulink Converter25/LConn1 -- Current Sensor25/RConn1
  Simulink-PS Converter13/RConn1 -- Switch13/RConn1
  R26/RConn1 -- D26/LConn1
  R28/RConn1 -- D28/LConn1
  Simulink-PS Converter16/RConn1 -- Switch16/RConn1
  Switch18/LConn1 -- D29/RConn1
  Current Sensor35/RConn2 -- R26/LConn1
  R33/RConn1 -- D33/LConn1
  Current Sensor28/RConn1 -- PS-Simulink Converter30/LConn1
  Current Sensor24/RConn2 -- R25/LConn1
  Current Sensor32/RConn1 -- PS-Simulink Converter34/LConn1
  Current Sensor28/RConn2 -- R29/LConn1
  R34/RConn1 -- D34/LConn1
  Switch19/LConn1 -- D30/RConn1
  Simulink-PS Converter24/RConn1 -- Switch36/RConn1
  Switch21/LConn1 -- D32/RConn1
  Switch15/LConn1 -- D27/RConn1
  Current Sensor33/RConn2 -- R35/LConn1
  R29/RConn1 -- D29/LConn1
  Current Sensor29/RConn1 -- PS-Simulink Converter31/LConn1
  Current Sensor35/RConn1 -- PS-Simulink Converter26/LConn1
  Current Sensor25/RConn2 -- R34/LConn1
  Current Sensor36/LConn1 -- Switch37/RConn2 -- Simscape Bus/LConn2
  Switch38/LConn1 -- D37/RConn1
  R38/RConn1 -- D38/LConn1
  PS-Simulink Converter37/LConn1 -- Current Sensor37/RConn1
  R37/RConn1 -- D37/LConn1
  Current Sensor36/RConn2 -- R37/LConn1
  Switch37/LConn1 -- D38/RConn1
  Current Sensor37/LConn1 -- Simscape Bus/LConn1
  Simulink-PS Converter26/RConn1 -- Switch38/RConn1
  PS-Simulink Converter38/LConn1 -- Current Sensor36/RConn1
  Simulink-PS Converter25/RConn1 -- Switch37/RConn1
  Current Sensor37/RConn2 -- R38/LConn1
